simulink model "Simulation_NoVI"  (R2022b)
settings: Solver=VariableStepAuto  StartTime=0.0  StopTime=25  RelTol=1e-3
values from neighbouring files (symbols this model uses):
  A = [0 1 1 1 ; 1 0 1 1 ; 1 1 0 1 ; 1 1 1 0]    [Primary_test1.m]    (also in init.mat = [0 1 1 1 1 0 1 1 1 1 0 1 ... (16 elements, 4x4)])
  C_f = 0.000112315*9    (= 0.001010835)    [Main.m]    (also in PSO_2paras.m = swarm(i,2); PSO_filter_2paras.m = swarm(i,2)/10000; Primary_test1.m; Script_18June.m = 0.0112315)
  f_c = 50e3    (= 50000)    [Main.m]    (also in Primary_test1.m; Script_18June.m; Script_23June.m; Script_5thJune.m)
  k = -0.5    [Main.m]    (also in Primary_test1.m; Savedata.m = 0.2909; Script_18June.m = 0.5; Script_23June.m)
  K_h11 = 0    [Main.m]    (also in PSO_HC.m = swarm(i,4); Primary_test1.m; Script_18June.m; Script_23June.m)
  K_h13 = 0    [Main.m]    (also in Primary_test1.m; Script_18June.m; Script_23June.m; Script_5thJune.m)
  K_h5 = 0    [Main.m]    (also in PSO_HC.m = swarm(i,1); Primary_test1.m = 1; Script_18June.m; Script_23June.m)
  K_h7 = 0    [Main.m]    (also in PSO_HC.m = swarm(i,2); Primary_test1.m; Script_18June.m; Script_23June.m)
  K_h9 = 0    [Main.m]    (also in PSO_HC.m = swarm(i,3); Script_18June.m; Script_23June.m; Script_5thJune.m)
  ki_pr = 160    [Main.m]    (also in PSO.m = swarm(i,2); Primary_test1.m; Savedata.m = 422.4716; Script_18June.m = 150)
  kL = 1e-7    (= 1e-07)    [Main.m]    (also in Primary_test1.m; Script_18June.m; Script_23June.m; Script_5thJune.m)
  Kp_pr = 1.7    [Main.m]    (also in PSO.m = swarm(i,1); Primary_test1.m; Savedata.m = 0.9028; Script_18June.m = 1)
  L_f = 0.000659829*1.4    (= 0.0009237606)    [Main.m]    (also in PSO_2paras.m = swarm(i,1); PSO_filter_2paras.m = swarm(i,1); Primary_test1.m; Script_18June.m = 0.000295603392)
  L_in1 = 0.35e-3    (= 0.00035)    [Main.m]    (also in Primary_test1.m; Script_18June.m; Script_23June.m; Script_5thJune.m)
  L_in2 = 0.35e-3    (= 0.00035)    [Main.m]    (also in Primary_test1.m; Script_18June.m; Script_23June.m; Script_5thJune.m)
  L_in3 = 0.35e-3    (= 0.00035)    [Main.m]    (also in Primary_test1.m; Script_18June.m; Script_23June.m; Script_5thJune.m)
  L_in4 = 0.35e-3    (= 0.00035)    [Main.m]    (also in Primary_test1.m; Script_18June.m; Script_23June.m; Script_5thJune.m)
  lambda1 = 5.5*[1 1 0.8 0.8]'    [Primary_test1.m]    (also in init.mat = [5.5 5.5 4.4 4.4])
  lambda2 = 30.5*[0.8e-2 0.8e-2 0.5e-2 0.5e-2]'    [Primary_test1.m]    (also in init.mat = [0.244 0.244 0.1525 0.1525])
  lambda3 = 62.5*[1.5e-3 1.5e-3 1e-3 1.1e-3]'    [Primary_test1.m]    (also in init.mat = [0.09375 0.09375 0.0625 0.06875])
  LD_ref1 = 100e-6    (= 0.0001)    [Main.m]    (also in Primary_test1.m; Script_18June.m = 5e-05; Script_23June.m = 1e-05; Script_5thJune.m = 1e-05)
  lo_co = 0.1    [Main.m]    (also in Primary_test1.m; Script_18June.m; Script_23June.m; Script_5thJune.m)
  load_off = 10    [Main.m]    (also in Primary_test1.m = 2; Script_18June.m = 28; Script_23June.m = 28; Script_5thJune.m)
  load_on = 0.21    [Main.m]    (also in Primary_test1.m = 1; Script_18June.m; Script_23June.m; Script_5thJune.m)
  m_p1 = 9.4e-5/droopDivide    (= 9.4e-06)    [Main.m]    (also in Primary_test1.m; Script_18June.m = 9.4e-05; Script_23June.m = 9.4e-05; Script_5thJune.m = 5e-05)
  m_p2 = 9.4e-5/droopDivide    (= 9.4e-06)    [Main.m]    (also in Primary_test1.m; Script_18June.m = 9.4e-05; Script_23June.m = 9.4e-05; Script_5thJune.m = 5e-05)
  m_p3 = 11.4e-5/droopDivide    (= 1.14e-05)    [Main.m]    (also in Primary_test1.m; Script_18June.m = 0.000114; Script_23June.m = 0.000114; Script_5thJune.m = 6.42857142857e-05)
  m_p4 = 11.4e-5/droopDivide    (= 1.14e-05)    [Main.m]    (also in Primary_test1.m; Script_18June.m = 0.000114; Script_23June.m = 0.000114; Script_5thJune.m = 6.42857142857e-05)
  N = 2    [Primary_test1.m]    (also in init.mat)
  n_q1 = 1.3e-3/droopDivide2    (= 6.5e-05)    [Main.m]    (also in Primary_test1.m; Script_18June.m; Script_23June.m; Script_5thJune.m = 0.2)
  n_q2 = 1.3e-3/droopDivide2    (= 6.5e-05)    [Main.m]    (also in Primary_test1.m; Script_18June.m; Script_23June.m; Script_5thJune.m = 0.2)
  n_q3 = 1.5e-3/droopDivide2    (= 7.5e-05)    [Main.m]    (also in Primary_test1.m; Script_18June.m; Script_23June.m; Script_5thJune.m = 0.257142857143)
  n_q4 = 1.5e-3/droopDivide2    (= 7.5e-05)    [Main.m]    (also in Primary_test1.m; Script_18June.m; Script_23June.m; Script_5thJune.m = 0.257142857143)
  Pmax = [45e3 45e3 37e3 37e3]'    [Primary_test1.m]    (also in init.mat = [45000 45000 37000 37000])
  PMW = V_nom/0.55    [Main.m]    (also in Primary_test1.m; Script_18June.m = V_nom/0.4; Script_23June.m; Script_5thJune.m = 220*sqrt(2))
  R_f = 0.35    [Main.m]    (also in PSO_filter_2paras.m = 10*L_f; Primary_test1.m; Savedata.m = 0.249593207053; Script_18June.m = 0.1)
  R_in1 = 0.03    [Main.m]    (also in Primary_test1.m; Script_18June.m; Script_23June.m; Script_5thJune.m)
  R_in2 = 0.03    [Main.m]    (also in Primary_test1.m; Script_18June.m; Script_23June.m; Script_5thJune.m)
  R_in3 = 0.03    [Main.m]    (also in Primary_test1.m; Script_18June.m; Script_23June.m; Script_5thJune.m)
  R_in4 = 0.03    [Main.m]    (also in Primary_test1.m; Script_18June.m; Script_23June.m; Script_5thJune.m)
  time_thresh = 0.2    [Main.m]    (also in Primary_test1.m; Script_18June.m; Script_23June.m; Script_5thJune.m)
  Ts = 10e-6    (= 1e-05)    [Main.m]    (also in Primary_test1.m; Script_18June.m; Script_23June.m; Script_5thJune.m)
  Tsamp = 0.1    [Primary_test1.m]    (also in init.mat)
  V_nom = 220*sqrt(2)    [Main.m]    (also in Primary_test1.m; Script_18June.m; Script_23June.m; Script_5thJune.m)
  Vdc = 600    [Main.m]    (also in Primary_test1.m; Script_18June.m; Script_23June.m; Script_5thJune.m)
  w_c_high = 2*pi*50    (= 314.159265359)    [Main.m]    (also in Primary_test1.m; Script_18June.m = 307.876080052; Script_23June.m; Script_5thJune.m = 307.876080052)
  w_nom = 2*pi*f    (= 314.159265359)    [Main.m]    (also in Primary_test1.m; Script_18June.m; Script_23June.m; Script_5thJune.m)
  wc_hc = 1    [Main.m]    (also in Primary_test1.m; Script_18June.m = 0.3; Script_23June.m; Script_5thJune.m = 0.3)
  wc_pr = 3    [Main.m]    (also in PSO.m = swarm(i,3); Primary_test1.m; Savedata.m = 1.36672; Script_18June.m = 1.5)
undefined symbols (not defined in the file or in its folder): DiscIntNeverNeededParam, i
libraries: eeGeneralControl x16, spsThreePhaseSeriesRLCBranchLib x15, spsThreePhaseVIMeasurementLib x12, spsabctoAlphaBetaZeroLib x12, spsabctodq0Lib x12, slpidlib x8, spsThreePhaseSeriesRLCLoadLib x6, spsThreePhaseBreakerLib x6, spsDCVoltageSourceLib x4, spsAlphaBetaZerotoabcLib x4, spsSeriesRLCBranchLib x4, spsTriangleGeneratorLib x4
(part 3 of 5)

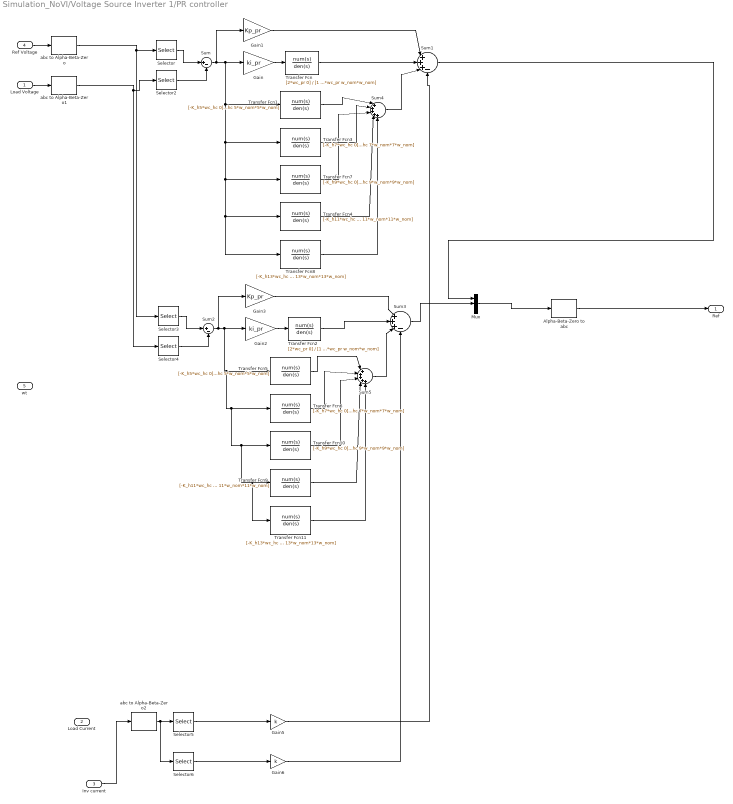
== system Simulation_NoVI/Voltage Source Inverter 1/PR controller ==
  Load Voltage : Inport
  Load Current : Inport  Port=2
  Inv current : Inport  Port=3
  Ref Voltage : Inport  Port=4
  wt : Inport  Port=5
  Alpha-Beta-Zero to abc : spsAlphaBetaZerotoabcLib/Alpha-Beta-Zero to abc
      settings: LibrarySourceBlock=|
      | sps_lib/Control/Alpha-Beta-Zero
      | to abc
  Gain : Gain  Gain=ki_pr
  Gain1 : Gain  Gain=Kp_pr
  Gain2 : Gain  Gain=ki_pr
  Gain3 : Gain  Gain=Kp_pr
  Gain5 : Gain  Gain=k
  Gain6 : Gain  Gain=k
  Mux : Mux  Inputs=3
  Selector : Selector  InputPortWidth=3  IndexOptions=Index vector (dialog)  Indices=[1]  OutputSizes=1
  Selector2 : Selector  InputPortWidth=3  IndexOptions=Index vector (dialog)  Indices=[1]  OutputSizes=1
  Selector3 : Selector  InputPortWidth=3  IndexOptions=Index vector (dialog)  Indices=[2]  OutputSizes=1
  Selector4 : Selector  InputPortWidth=3  IndexOptions=Index vector (dialog)  Indices=[2]  OutputSizes=1
  Selector5 : Selector  InputPortWidth=3  IndexOptions=Index vector (dialog)  Indices=[1]  OutputSizes=1
  Selector6 : Selector  InputPortWidth=3  IndexOptions=Index vector (dialog)  Indices=[2]  OutputSizes=1
  Sum : Sum  Inputs=|+-
  Sum1 : Sum  Inputs=|+++-
  Sum2 : Sum  Inputs=|+-
  Sum3 : Sum  Inputs=|+++-
  Sum4 : Sum  Inputs=|+++++
  Sum5 : Sum  Inputs=|+++++
  Transfer Fcn : TransferFcn  Numerator=[2*wc_pr 0]  Denominator=[1 2*wc_pr*wc_pr w_nom*w_nom]
  Transfer Fcn1 : TransferFcn  Numerator=[-K_h5*wc_hc 0]  Denominator=[1 2*wc_hc 5*w_nom*5*w_nom]
  Transfer Fcn10 : TransferFcn  Numerator=[-K_h9*wc_hc 0]  Denominator=[1 2*wc_hc 9*w_nom*9*w_nom]
  Transfer Fcn11 : TransferFcn  Numerator=[-K_h13*wc_hc 0]  Denominator=[1 2*wc_hc 13*w_nom*13*w_nom]
  Transfer Fcn2 : TransferFcn  Numerator=[2*wc_pr 0]  Denominator=[1 2*wc_pr*wc_pr w_nom*w_nom]
  Transfer Fcn3 : TransferFcn  Numerator=[-K_h7*wc_hc 0]  Denominator=[1 2*wc_hc 7*w_nom*7*w_nom]
  Transfer Fcn4 : TransferFcn  Numerator=[-K_h11*wc_hc 0]  Denominator=[1 2*wc_hc 11*w_nom*11*w_nom]
  Transfer Fcn5 : TransferFcn  Numerator=[-K_h5*wc_hc 0]  Denominator=[1 2*wc_hc 5*w_nom*5*w_nom]
  Transfer Fcn6 : TransferFcn  Numerator=[-K_h7*wc_hc 0]  Denominator=[1 2*wc_hc 7*w_nom*7*w_nom]
  Transfer Fcn7 : TransferFcn  Numerator=[-K_h9*wc_hc 0]  Denominator=[1 2*wc_hc 9*w_nom*9*w_nom]
  Transfer Fcn8 : TransferFcn  Numerator=[-K_h13*wc_hc 0]  Denominator=[1 2*wc_hc 13*w_nom*13*w_nom]
  Transfer Fcn9 : TransferFcn  Numerator=[-K_h11*wc_hc 0]  Denominator=[1 2*wc_hc 11*w_nom*11*w_nom]
  abc to Alpha-Beta-Zero : spsabctoAlphaBetaZeroLib/abc to Alpha-Beta-Zero
  abc to Alpha-Beta-Zero1 : spsabctoAlphaBetaZeroLib/abc to Alpha-Beta-Zero
  abc to Alpha-Beta-Zero2 : spsabctoAlphaBetaZeroLib/abc to Alpha-Beta-Zero
  Ref : Outport
  wires:
  Ref Voltage/1 -> abc to Alpha-Beta-Zero/1
  Selector/1 -> Sum/1
  Selector2/1 -> Sum/2
  Sum/1 -> Gain1/1, Transfer Fcn8/1, Transfer Fcn4/1, Transfer Fcn7/1, Transfer Fcn3/1, Transfer Fcn1/1, Gain/1
  Gain/1 -> Transfer Fcn/1
  Gain1/1 -> Sum1/1
  Transfer Fcn/1 -> Sum1/2
  Sum2/1 -> Gain3/1, Transfer Fcn11/1, Transfer Fcn9/1, Transfer Fcn10/1, Transfer Fcn6/1, Transfer Fcn5/1, Gain2/1
  Selector3/1 -> Sum2/1
  Gain2/1 -> Transfer Fcn2/1
  Transfer Fcn2/1 -> Sum3/2
  Gain3/1 -> Sum3/1
  abc to Alpha-Beta-Zero2/1 -> Selector6/1, Selector5/1
  Sum1/1 -> Mux/1
  Sum3/1 -> Mux/2
  Mux/1 -> Alpha-Beta-Zero to abc/1
  Inv current/1 -> abc to Alpha-Beta-Zero2/1
  Sum4/1 -> Sum1/3
  Transfer Fcn1/1 -> Sum4/1
  Transfer Fcn3/1 -> Sum4/2
  Transfer Fcn6/1 -> Sum5/2
  Selector4/1 -> Sum2/2
  Sum5/1 -> Sum3/3
  Transfer Fcn7/1 -> Sum4/3
  Transfer Fcn4/1 -> Sum4/4
  Transfer Fcn8/1 -> Sum4/5
  Transfer Fcn10/1 -> Sum5/3
  Transfer Fcn9/1 -> Sum5/4
  Transfer Fcn11/1 -> Sum5/5
  Selector6/1 -> Gain6/1
  Selector5/1 -> Gain5/1
  Transfer Fcn5/1 -> Sum5/1
  Gain5/1 -> Sum1/4
  Gain6/1 -> Sum3/4
  Load Voltage/1 -> abc to Alpha-Beta-Zero1/1
  abc to Alpha-Beta-Zero/1 -> Selector3/1, Selector/1
  abc to Alpha-Beta-Zero1/1 -> Selector4/1, Selector2/1
  Alpha-Beta-Zero to abc/1 -> Ref/1

== system Simulation_NoVI/Voltage Source Inverter 1/dq converter ==
  Vodq : Inport
  Iodq : Inport  Port=2
  Ildq : Inport  Port=3
  wt : Inport  Port=4
  Scope : Scope
  Scope1 : Scope
  Subsystem : Subsystem
  Subsystem1 : Subsystem
  Subsystem2 : Subsystem
  Vod : Outport
  Voq : Outport  Port=2
  Iod : Outport  Port=3
  Ioq : Outport  Port=4
  Ild : Outport  Port=5
  Ilq : Outport  Port=6
  wires:
  Subsystem/1(Out1) -> Scope/1, Vod/1  "Vod"
  Subsystem1/1(Out1) -> Iod/1  "Iod"
  Subsystem/2(Out2) -> Voq/1  "Voq"
  wt/1 -> Subsystem2/2(wt), Subsystem1/2(wt), Subsystem/2(wt)
  Subsystem1/2(Out2) -> Ioq/1  "Ioq"
  Iodq/1 -> Subsystem1/1(abc)
  Subsystem2/2(Out2) -> Ilq/1  "Ilq"
  Ildq/1 -> Subsystem2/1(abc)
  Vodq/1 -> Subsystem/1(abc)
  Subsystem2/1(Out1) -> Scope1/1, Ild/1  "Vod"

== system Simulation_NoVI/Voltage Source Inverter 2/3to2 3 ==
  "single " : Inport
  "wt " : Inport  Port=2
  Add1 : Sum  Inputs=+++
  Constant2 : Constant  Value=2*pi/3
  Constant3 : Constant  Value=4*pi/3
  Constant4 : Constant  Value=exp(i*2*pi/3)
  Constant5 : Constant  Value=2/3
  Cos : Trigonometry  Operator=cos
  Cos1 : Trigonometry  Operator=cos
  Cos2 : Trigonometry  Operator=cos
  Math Function1 : Math  Operator=square  SignedPower=on
  Mux : Mux  Inputs=3
  Product{3..8} (6 alike) : Product  RndMeth=Zero
  Scope : Scope  NumInputPorts=3
  Sum : Sum  Inputs=|++
  Sum1 : Sum  Inputs=|++
  threePhase : Outport  VectorParamsAs1DForOutWhenUnconnected=off
  wires:
  "single "/1 -> Product5/1, Product4/1, Product3/1
  Cos/1 -> Product3/2
  Constant2/1 -> Sum/2
  Sum/1 -> Cos1/1
  Cos1/1 -> Product4/2
  "wt "/1 -> Sum1/1, Sum/1, Cos/1
  Constant3/1 -> Sum1/2
  Sum1/1 -> Cos2/1
  Cos2/1 -> Product5/2
  Constant4/1 -> Product7/1, Math Function1/1
  Product7/1 -> Add1/2
  Add1/1 -> Product6/1
  Product8/1 -> Add1/3
  Product5/1 -> Scope/3, Mux/3, Product8/2
  Product3/1 -> Scope/1, Mux/1, Add1/1
  Constant5/1 -> Product6/2
  Product4/1 -> Scope/2, Mux/2, Product7/2
  Math Function1/1 -> Product8/1
  Mux/1 -> threePhase/1

== system Simulation_NoVI/Voltage Source Inverter 2/Droop for secondary control2 ==
  P : Inport
  w_nom : Inport  Port=2
  V_nom : Inport  Port=3
  Q : Inport  Port=4
  Gain4 : Gain  Gain=n_q
  Gain5 : Gain  Gain=m_p
  Integrator : Integrator  WrapState=on  WrappedStateUpperValue=2*pi  WrappedStateLowerValue=0
  Sum1 : Sum  Inputs=|+-
  Sum2 : Sum  Inputs=|+-
  Vref : Outport
  wt : Outport  Port=2
  wo : Outport  Port=3
  wires:
  P/1 -> Gain5/1
  w_nom/1 -> Sum2/1
  Gain5/1 -> Sum2/2
  Sum2/1 -> wo/1, Integrator/1  "w"
  Integrator/1 -> wt/1
  V_nom/1 -> Sum1/1  "Vod_s"
  Gain4/1 -> Sum1/2
  Q/1 -> Gain4/1
  Sum1/1 -> Vref/1  "Vod_s"

== system Simulation_NoVI/Voltage Source Inverter 2/Low-pass filter ==
  p_hat : Inport
  q_hat : Inport  Port=2
  Low-Pass Filter (Discrete or Continuous) : eeGeneralControl/Low-Pass Filter (Discrete or Continuous)  K=1  T=lo_co  B=inf  A=-inf  init_option=Inherited from block input  x0=0  Ts=-1
  Low-Pass Filter (Discrete or Continuous)1 : eeGeneralControl/Low-Pass Filter (Discrete or Continuous)  K=1  T=lo_co  B=inf  A=-inf  init_option=Inherited from block input  x0=0  Ts=-1
  P : Outport
  Q : Outport  Port=2
  wires:
  q_hat/1 -> Low-Pass Filter (Discrete or Continuous)1/1
  Low-Pass Filter (Discrete or Continuous)1/1 -> Q/1  "Q"
  Low-Pass Filter (Discrete or Continuous)/1 -> P/1  "P"
  p_hat/1 -> Low-Pass Filter (Discrete or Continuous)/1

== system Simulation_NoVI/Voltage Source Inverter 2/PLL_1p1 ==
  v : Inport
  2pi : Constant  Value=2*pi
  Low-Pass Filter (Discrete or Continuous) : eeGeneralControl/Low-Pass Filter (Discrete or Continuous)  K=1  T=lo_co  B=inf  A=-inf  init_option=Inherited from block input  x0=0  Ts=-1
  PID Controller : slpidlib/PID Controller  Controller=PI  Form=Parallel  TimeDomain=Continuous-time  UseExternalTs=off  SampleTime=-1  IntegratorMethod=Forward Euler  FilterMethod=Forward Euler  ControllerParametersSource=internal  P=100.15925  I=9869  UseKiTs=off  D=0  N=100  UseFilter=on  TunerSelectOption=Transfer Function Based (PID Tuner App)  InitialConditionSource=internal  InitialConditionForIntegrator=0  InitialConditionForFilter=0  DifferentiatorICPrevScaledInput=0  ExternalReset=none  TrackingMode=off  Kt=1  LimitOutput=off  SatLimitsSource=internal  UpperSaturationLimit=inf  LowerSaturationLimit=-inf  LinearizeAsGain=off  AntiWindupMode=none  Kb=1  LimitIntegrator=off  UpperIntegratorSaturationLimit=inf  LowerIntegratorSaturationLimit=-inf  POutMin=[]  POutMax=[]  IOutMin=[]  IOutMax=[]  DOutMin=[]  DOutMax=[]  NOutMin=[]  NOutMax=[]  SumOutMin=[]  SumOutMax=[]  SaturationOutMin=[]  SaturationOutMax=[]  PParamMin=[]  PParamMax=[]  IParamMin=[]  IParamMax=[]  DParamMin=[]  DParamMax=[]  NParamMin=[]  NParamMax=[]  KbParamMin=[]  KbParamMax=[]  KtParamMin=[]  KtParamMax=[]  KbOutMin=[]  KbOutMax=[]  KtOutMin=[]  KtOutMax=[]  IntegratorOutMin=[]  IntegratorOutMax=[]  FilterOutMin=[]  FilterOutMax=[]  SumI1OutMin=[]  SumI1OutMax=[]  SumI2OutMin=[]  SumI2OutMax=[]  SumI3OutMin=[]  SumI3OutMax=[]  SumI4OutMin=[]  SumI4OutMax=[]  SumDOutMin=[]  SumDOutMax=[]  DifferentiatorOutMin=[]  DifferentiatorOutMax=[]  FilterDiffOutCoefMin=[]  FilterDiffOutCoefMax=[]  ReciprocalOutMin=[]  ReciprocalOutMax=[]  SumDenOutMin=[]  SumDenOutMax=[]  SumNumOutMin=[]  SumNumOutMax=[]  DivideOutMin=[]  DivideOutMax=[]  UdiffTsProdOutMin=[]  UdiffTsProdOutMax=[]  NTsProdOutMin=[]  NTsProdOutMax=[]  UintegralTsProdOutMin=[]  UintegralTsProdOutMax=[]  UngainTsProdOutMin=[]  UngainTsProdOutMax=[]  ClampingZeroOutDataTypeStr=Inherit: Inherit via back propagation  ClampingZeroOutMin=[]  ClampingZeroOutMax=[]  FilterDenConstantOutDataTypeStr=Inherit: Inherit via back propagation  FilterDenConstantOutMin=[]  FilterDenConstantOutMax=[]  PCopyOutDataTypeStr=Inherit: Inherit via back propagation  PCopyOutMin=[]  PCopyOutMax=[]  NCopyOutDataTypeStr=Inherit: Inherit via back propagation  NCopyOutMin=[]  NCopyOutMax=[]  IntegratorContinuousStateAttributes=''  IntegratorStateMustResolveToSignalObject=off  IntegratorRTWStateStorageClass=Auto  FilterContinuousStateAttributes=''  FilterStateMustResolveToSignalObject=off  FilterRTWStateStorageClass=Auto  ParallelPVariant=InternalParameters  IdealPVariant=Disabled  IVariant=InternalParameters  DVariant=Disabled  IntegratorVariant=Continuous  SatVariant=Disabled  AWVariant=Passthrough  PCopyVariant=Disabled  TRVariant=Disabled  FdbkBlocksVariant=Forward  IdealPFdbkVariant=Disabled  SatFdbkVariant=Disabled  DerivativeFilterVariant=Disabled  NVariant=Disabled  NCopyVariant=Disabled_SignalSpec  FilterICVariant=Disabled  IntegratorICVariant=InternalICs  ExternalResetVariant=Disabled  TRSumVariant=Passthrough  SumFdbkVariant=Disabled  SumVariant=Sum_PI  TsampFilterVariant=InternalTs  TsampNgainVariant=Passthrough  TsampIntegralVariant=Passthrough  ExternalSaturationOutDataTypeStr=Inherit: Same as second input
  Reset1 : RelationalOperator  OutDataTypeStr=boolean  InputSameDT=off
  Scope : Scope
  Sqrt : Sqrt
  Square : Math  Operator=square
  Square1 : Math  Operator=square
  Sum : Sum  Inputs=|++
  Sum1 : Sum  Inputs=|++
  TienXuly : Subsystem  mask{k=0.5, fc1=50, fc2=10}
      mask prompts: k "he so k"; fc1 "Tan so cat cua bo loc bac 2"; fc2 "Tan so cat cua bo loc thong thap"
  Tinhtheta : Integrator  ExternalReset=rising  UpperSaturationLimit=2*pi
  apha-beta=>dq : Subsystem
  wff : Constant  Value=50*2*pi
  v_dq : Outport
  omega : Outport  Port=2
  wires:
  PID Controller/1 -> Sum1/1
  v/1 -> TienXuly/1(v)
  Tinhtheta/1 -> apha-beta=>dq/1(Theta), Reset1/1
  TienXuly/2(v'q) -> apha-beta=>dq/3(Ubeta)
  apha-beta=>dq/1(vq) -> Square1/1, PID Controller/1
  TienXuly/1(v') -> apha-beta=>dq/2(Uapha)
  2pi/1 -> Reset1/2
  wff/1 -> Sum1/2
  Reset1/1 -> Tinhtheta/2
  apha-beta=>dq/2(vd) -> Square/1
  Square/1 -> Sum/1
  Square1/1 -> Sum/2
  Sum/1 -> Sqrt/1
  Sqrt/1 -> v_dq/1
  Sum1/1 -> Low-Pass Filter (Discrete or Continuous)/1, Tinhtheta/1  "P"
  Low-Pass Filter (Discrete or Continuous)/1 -> Scope/1, omega/1  "P"

== system Simulation_NoVI/Voltage Source Inverter 2/PLL_1p2 ==
  v : Inport
  2pi : Constant  Value=2*pi
  Low-Pass Filter (Discrete or Continuous) : eeGeneralControl/Low-Pass Filter (Discrete or Continuous)  K=1  T=lo_co  B=inf  A=-inf  init_option=Inherited from block input  x0=0  Ts=-1
  PID Controller : slpidlib/PID Controller  Controller=PI  Form=Parallel  TimeDomain=Continuous-time  UseExternalTs=off  SampleTime=-1  IntegratorMethod=Forward Euler  FilterMethod=Forward Euler  ControllerParametersSource=internal  P=100.15925  I=9869  UseKiTs=off  D=0  N=100  UseFilter=on  TunerSelectOption=Transfer Function Based (PID Tuner App)  InitialConditionSource=internal  InitialConditionForIntegrator=0  InitialConditionForFilter=0  DifferentiatorICPrevScaledInput=0  ExternalReset=none  TrackingMode=off  Kt=1  LimitOutput=off  SatLimitsSource=internal  UpperSaturationLimit=inf  LowerSaturationLimit=-inf  LinearizeAsGain=off  AntiWindupMode=none  Kb=1  LimitIntegrator=off  UpperIntegratorSaturationLimit=inf  LowerIntegratorSaturationLimit=-inf  POutMin=[]  POutMax=[]  IOutMin=[]  IOutMax=[]  DOutMin=[]  DOutMax=[]  NOutMin=[]  NOutMax=[]  SumOutMin=[]  SumOutMax=[]  SaturationOutMin=[]  SaturationOutMax=[]  PParamMin=[]  PParamMax=[]  IParamMin=[]  IParamMax=[]  DParamMin=[]  DParamMax=[]  NParamMin=[]  NParamMax=[]  KbParamMin=[]  KbParamMax=[]  KtParamMin=[]  KtParamMax=[]  KbOutMin=[]  KbOutMax=[]  KtOutMin=[]  KtOutMax=[]  IntegratorOutMin=[]  IntegratorOutMax=[]  FilterOutMin=[]  FilterOutMax=[]  SumI1OutMin=[]  SumI1OutMax=[]  SumI2OutMin=[]  SumI2OutMax=[]  SumI3OutMin=[]  SumI3OutMax=[]  SumI4OutMin=[]  SumI4OutMax=[]  SumDOutMin=[]  SumDOutMax=[]  DifferentiatorOutMin=[]  DifferentiatorOutMax=[]  FilterDiffOutCoefMin=[]  FilterDiffOutCoefMax=[]  ReciprocalOutMin=[]  ReciprocalOutMax=[]  SumDenOutMin=[]  SumDenOutMax=[]  SumNumOutMin=[]  SumNumOutMax=[]  DivideOutMin=[]  DivideOutMax=[]  UdiffTsProdOutMin=[]  UdiffTsProdOutMax=[]  NTsProdOutMin=[]  NTsProdOutMax=[]  UintegralTsProdOutMin=[]  UintegralTsProdOutMax=[]  UngainTsProdOutMin=[]  UngainTsProdOutMax=[]  ClampingZeroOutDataTypeStr=Inherit: Inherit via back propagation  ClampingZeroOutMin=[]  ClampingZeroOutMax=[]  FilterDenConstantOutDataTypeStr=Inherit: Inherit via back propagation  FilterDenConstantOutMin=[]  FilterDenConstantOutMax=[]  PCopyOutDataTypeStr=Inherit: Inherit via back propagation  PCopyOutMin=[]  PCopyOutMax=[]  NCopyOutDataTypeStr=Inherit: Inherit via back propagation  NCopyOutMin=[]  NCopyOutMax=[]  IntegratorContinuousStateAttributes=''  IntegratorStateMustResolveToSignalObject=off  IntegratorRTWStateStorageClass=Auto  FilterContinuousStateAttributes=''  FilterStateMustResolveToSignalObject=off  FilterRTWStateStorageClass=Auto  ParallelPVariant=InternalParameters  IdealPVariant=Disabled  IVariant=InternalParameters  DVariant=Disabled  IntegratorVariant=Continuous  SatVariant=Disabled  AWVariant=Passthrough  PCopyVariant=Disabled  TRVariant=Disabled  FdbkBlocksVariant=Forward  IdealPFdbkVariant=Disabled  SatFdbkVariant=Disabled  DerivativeFilterVariant=Disabled  NVariant=Disabled  NCopyVariant=Disabled_SignalSpec  FilterICVariant=Disabled  IntegratorICVariant=InternalICs  ExternalResetVariant=Disabled  TRSumVariant=Passthrough  SumFdbkVariant=Disabled  SumVariant=Sum_PI  TsampFilterVariant=InternalTs  TsampNgainVariant=Passthrough  TsampIntegralVariant=Passthrough  ExternalSaturationOutDataTypeStr=Inherit: Same as second input
  Reset1 : RelationalOperator  OutDataTypeStr=boolean  InputSameDT=off
  Scope : Scope
  Sqrt : Sqrt
  Square : Math  Operator=square
  Square1 : Math  Operator=square
  Sum : Sum  Inputs=|++
  Sum1 : Sum  Inputs=|++
  TienXuly : Subsystem  mask{k=0.5, fc1=50, fc2=10}
      mask prompts: k "he so k"; fc1 "Tan so cat cua bo loc bac 2"; fc2 "Tan so cat cua bo loc thong thap"
  Tinhtheta : Integrator  ExternalReset=rising  UpperSaturationLimit=2*pi
  apha-beta=>dq : Subsystem
  wff : Constant  Value=50*2*pi
  v_dq : Outport
  omega : Outport  Port=2
  wires:
  PID Controller/1 -> Sum1/1
  v/1 -> TienXuly/1(v)
  Tinhtheta/1 -> apha-beta=>dq/1(Theta), Reset1/1
  TienXuly/2(v'q) -> apha-beta=>dq/3(Ubeta)
  apha-beta=>dq/1(vq) -> Square1/1, PID Controller/1
  TienXuly/1(v') -> apha-beta=>dq/2(Uapha)
  2pi/1 -> Reset1/2
  wff/1 -> Sum1/2
  Reset1/1 -> Tinhtheta/2
  apha-beta=>dq/2(vd) -> Square/1
  Square/1 -> Sum/1
  Square1/1 -> Sum/2
  Sum/1 -> Sqrt/1
  Sqrt/1 -> v_dq/1
  Sum1/1 -> Low-Pass Filter (Discrete or Continuous)/1, Tinhtheta/1  "P"
  Low-Pass Filter (Discrete or Continuous)/1 -> Scope/1, omega/1  "P"

== system Simulation_NoVI/Voltage Source Inverter 2/PMW ==
  REF : Inport
  Tri_signal : Inport  Port=2
  Demux : Demux  Outputs=3
  Mux : Mux  Inputs=6
  NOT : Logic  Operator=NOT  AllPortsSameDT=off  OutDataTypeStr=boolean
  NOT1 : Logic  Operator=NOT  AllPortsSameDT=off  OutDataTypeStr=boolean
  NOT2 : Logic  Operator=NOT  AllPortsSameDT=off  OutDataTypeStr=boolean
  Relational Operator : RelationalOperator  OutDataTypeStr=boolean  RndMeth=Simplest  InputSameDT=off
  Relational Operator1 : RelationalOperator  OutDataTypeStr=boolean  RndMeth=Simplest  InputSameDT=off
  Relational Operator2 : RelationalOperator  OutDataTypeStr=boolean  RndMeth=Simplest  InputSameDT=off
  Scope : Scope
  Scope1 : Scope
  Scope2 : Scope  NumInputPorts=2
  Out1 : Outport
  wires:
  Demux/1 -> Relational Operator/1
  Tri_signal/1 -> Relational Operator1/2, Relational Operator/2, Relational Operator2/2
  Demux/2 -> Relational Operator1/1
  Demux/3 -> Relational Operator2/1
  REF/1 -> Scope1/1, Demux/1
  Relational Operator/1 -> Scope2/1, Mux/1, NOT/1
  NOT/1 -> Scope2/2, Mux/2
  Relational Operator1/1 -> NOT1/1, Mux/3
  NOT1/1 -> Mux/4
  Relational Operator2/1 -> Mux/5, NOT2/1
  NOT2/1 -> Mux/6
  Mux/1 -> Scope/1, Out1/1

== system Simulation_NoVI/Voltage Source Inverter 2/PQ calculator ==
  Vod : Inport
  Voq : Inport  Port=2
  Iod : Inport  Port=3
  Ioq : Inport  Port=4
  Product{,1..3} (4 alike) : Product
  Scope : Scope
  Sum10 : Sum  Inputs=|++
  Sum11 : Sum  Inputs=|+-
  p_hat : Outport
  q_hat : Outport  Port=2
  wires:
  Product3/1 -> Sum11/2
  Product1/1 -> Sum10/2
  Voq/1 -> Product3/1, Product1/1
  Iod/1 -> Product/2, Product3/2
  Product2/1 -> Sum11/1
  Ioq/1 -> Product1/2, Product2/2
  Product/1 -> Sum10/1
  Vod/1 -> Scope/1, Product/1, Product2/1
  Sum11/1 -> q_hat/1  "q_hat"
  Sum10/1 -> p_hat/1  "p_hat"

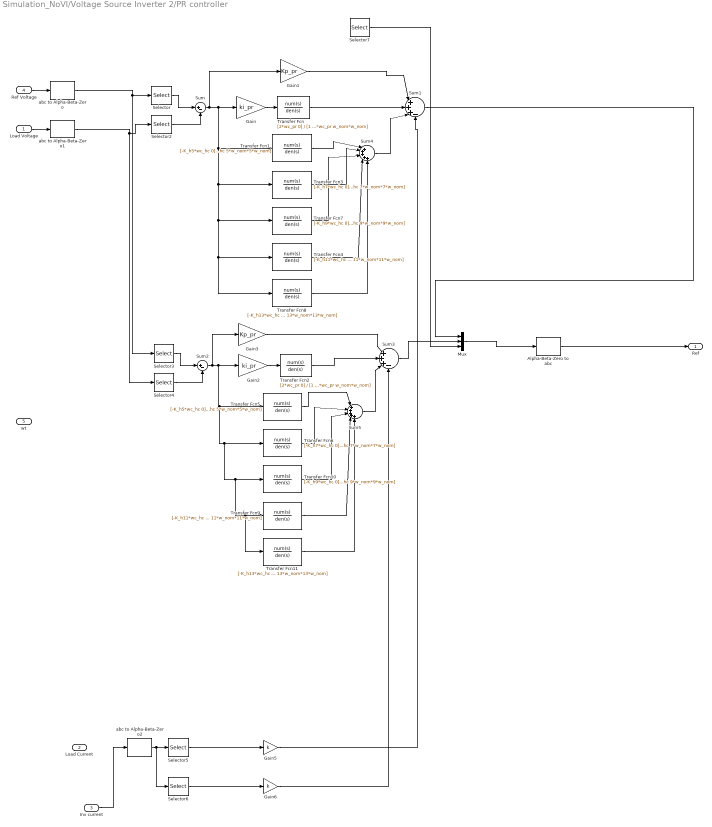
== system Simulation_NoVI/Voltage Source Inverter 2/PR controller ==
  Load Voltage : Inport
  Load Current : Inport  Port=2
  Inv current : Inport  Port=3
  Ref Voltage : Inport  Port=4
  wt : Inport  Port=5
  Alpha-Beta-Zero to abc : spsAlphaBetaZerotoabcLib/Alpha-Beta-Zero to abc
      settings: LibrarySourceBlock=|
      | sps_lib/Control/Alpha-Beta-Zero
      | to abc
  Gain : Gain  Gain=ki_pr
  Gain1 : Gain  Gain=Kp_pr
  Gain2 : Gain  Gain=ki_pr
  Gain3 : Gain  Gain=Kp_pr
  Gain5 : Gain  Gain=k
  Gain6 : Gain  Gain=k
  Mux : Mux  Inputs=3
  Selector : Selector  InputPortWidth=3  IndexOptions=Index vector (dialog)  Indices=[1]  OutputSizes=1
  Selector2 : Selector  InputPortWidth=3  IndexOptions=Index vector (dialog)  Indices=[1]  OutputSizes=1
  Selector3 : Selector  InputPortWidth=3  IndexOptions=Index vector (dialog)  Indices=[2]  OutputSizes=1
  Selector4 : Selector  InputPortWidth=3  IndexOptions=Index vector (dialog)  Indices=[2]  OutputSizes=1
  Selector5 : Selector  InputPortWidth=3  IndexOptions=Index vector (dialog)  Indices=[1]  OutputSizes=1
  Selector6 : Selector  InputPortWidth=3  IndexOptions=Index vector (dialog)  Indices=[2]  OutputSizes=1
  Selector7 : Selector  InputPortWidth=3  IndexOptions=Index vector (dialog)  Indices=[3]  OutputSizes=1
  Sum : Sum  Inputs=|+-
  Sum1 : Sum  Inputs=|+++-
  Sum2 : Sum  Inputs=|+-
  Sum3 : Sum  Inputs=|+++-
  Sum4 : Sum  Inputs=|+++++
  Sum5 : Sum  Inputs=|+++++
  Transfer Fcn : TransferFcn  Numerator=[2*wc_pr 0]  Denominator=[1 2*wc_pr*wc_pr w_nom*w_nom]
  Transfer Fcn1 : TransferFcn  Numerator=[-K_h5*wc_hc 0]  Denominator=[1 2*wc_hc 5*w_nom*5*w_nom]
  Transfer Fcn10 : TransferFcn  Numerator=[-K_h9*wc_hc 0]  Denominator=[1 2*wc_hc 9*w_nom*9*w_nom]
  Transfer Fcn11 : TransferFcn  Numerator=[-K_h13*wc_hc 0]  Denominator=[1 2*wc_hc 13*w_nom*13*w_nom]
  Transfer Fcn2 : TransferFcn  Numerator=[2*wc_pr 0]  Denominator=[1 2*wc_pr*wc_pr w_nom*w_nom]
  Transfer Fcn3 : TransferFcn  Numerator=[-K_h7*wc_hc 0]  Denominator=[1 2*wc_hc 7*w_nom*7*w_nom]
  Transfer Fcn4 : TransferFcn  Numerator=[-K_h11*wc_hc 0]  Denominator=[1 2*wc_hc 11*w_nom*11*w_nom]
  Transfer Fcn5 : TransferFcn  Numerator=[-K_h5*wc_hc 0]  Denominator=[1 2*wc_hc 5*w_nom*5*w_nom]
  Transfer Fcn6 : TransferFcn  Numerator=[-K_h7*wc_hc 0]  Denominator=[1 2*wc_hc 7*w_nom*7*w_nom]
  Transfer Fcn7 : TransferFcn  Numerator=[-K_h9*wc_hc 0]  Denominator=[1 2*wc_hc 9*w_nom*9*w_nom]
  Transfer Fcn8 : TransferFcn  Numerator=[-K_h13*wc_hc 0]  Denominator=[1 2*wc_hc 13*w_nom*13*w_nom]
  Transfer Fcn9 : TransferFcn  Numerator=[-K_h11*wc_hc 0]  Denominator=[1 2*wc_hc 11*w_nom*11*w_nom]
  abc to Alpha-Beta-Zero : spsabctoAlphaBetaZeroLib/abc to Alpha-Beta-Zero
  abc to Alpha-Beta-Zero1 : spsabctoAlphaBetaZeroLib/abc to Alpha-Beta-Zero
  abc to Alpha-Beta-Zero2 : spsabctoAlphaBetaZeroLib/abc to Alpha-Beta-Zero
  Ref : Outport
  wires:
  Ref Voltage/1 -> abc to Alpha-Beta-Zero/1
  Selector/1 -> Sum/1
  Selector2/1 -> Sum/2
  Sum/1 -> Gain1/1, Transfer Fcn8/1, Transfer Fcn4/1, Transfer Fcn7/1, Transfer Fcn3/1, Transfer Fcn1/1, Gain/1
  Gain/1 -> Transfer Fcn/1
  Gain1/1 -> Sum1/1
  Transfer Fcn/1 -> Sum1/2
  Sum2/1 -> Gain3/1, Transfer Fcn11/1, Transfer Fcn9/1, Transfer Fcn10/1, Transfer Fcn6/1, Transfer Fcn5/1, Gain2/1
  Selector3/1 -> Sum2/1
  Gain2/1 -> Transfer Fcn2/1
  Transfer Fcn2/1 -> Sum3/2
  Gain3/1 -> Sum3/1
  abc to Alpha-Beta-Zero2/1 -> Selector6/1, Selector5/1
  Sum1/1 -> Mux/1
  Sum3/1 -> Mux/2
  Mux/1 -> Alpha-Beta-Zero to abc/1
  Inv current/1 -> abc to Alpha-Beta-Zero2/1
  Sum4/1 -> Sum1/3
  Transfer Fcn1/1 -> Sum4/1
  Transfer Fcn3/1 -> Sum4/2
  Transfer Fcn6/1 -> Sum5/2
  Selector4/1 -> Sum2/2
  Sum5/1 -> Sum3/3
  Transfer Fcn7/1 -> Sum4/3
  Transfer Fcn4/1 -> Sum4/4
  Transfer Fcn8/1 -> Sum4/5
  Transfer Fcn10/1 -> Sum5/3
  Transfer Fcn9/1 -> Sum5/4
  Transfer Fcn11/1 -> Sum5/5
  Selector6/1 -> Gain6/1
  Selector5/1 -> Gain5/1
  Transfer Fcn5/1 -> Sum5/1
  Selector7/1 -> Mux/3
  Gain5/1 -> Sum1/4
  Gain6/1 -> Sum3/4
  Load Voltage/1 -> abc to Alpha-Beta-Zero1/1
  abc to Alpha-Beta-Zero/1 -> Selector3/1, Selector/1
  abc to Alpha-Beta-Zero1/1 -> Selector4/1, Selector2/1
  Alpha-Beta-Zero to abc/1 -> Ref/1

== system Simulation_NoVI/Voltage Source Inverter 2/THD measurement ==
  In1 : Inport
  Demux : Demux  Outputs=3
  To Workspace : ToWorkspace  VariableName=phase1  SaveFormat=Structure With Time  SampleTime=-1
  To Workspace1 : ToWorkspace  VariableName=phase2  SaveFormat=Structure With Time  SampleTime=-1
  To Workspace2 : ToWorkspace  VariableName=phase3  SaveFormat=Structure With Time  SampleTime=-1
  wires:
  In1/1 -> Demux/1
  Demux/1 -> To Workspace/1
  Demux/2 -> To Workspace1/1
  Demux/3 -> To Workspace2/1

== system Simulation_NoVI/Voltage Source Inverter 2/dq converter ==
  Vodq : Inport
  Iodq : Inport  Port=2
  Ildq : Inport  Port=3
  wt : Inport  Port=4
  Scope : Scope
  Scope1 : Scope
  Subsystem : Subsystem
  Subsystem1 : Subsystem
  Subsystem2 : Subsystem
  Vod : Outport
  Voq : Outport  Port=2
  Iod : Outport  Port=3
  Ioq : Outport  Port=4
  Ild : Outport  Port=5
  Ilq : Outport  Port=6
  wires:
  Subsystem/1(Out1) -> Scope/1, Vod/1  "Vod"
  Subsystem1/1(Out1) -> Iod/1  "Iod"
  Subsystem/2(Out2) -> Voq/1  "Voq"
  wt/1 -> Subsystem2/2(wt), Subsystem1/2(wt), Subsystem/2(wt)
  Subsystem1/2(Out2) -> Ioq/1  "Ioq"
  Iodq/1 -> Subsystem1/1(abc)
  Subsystem2/2(Out2) -> Ilq/1  "Ilq"
  Ildq/1 -> Subsystem2/1(abc)
  Vodq/1 -> Subsystem/1(abc)
  Subsystem2/1(Out1) -> Scope1/1, Ild/1  "Vod"

== system Simulation_NoVI/Voltage Source Inverter 3/3to2 3 ==
  "single " : Inport
  "wt " : Inport  Port=2
  Add1 : Sum  Inputs=+++
  Constant2 : Constant  Value=2*pi/3
  Constant3 : Constant  Value=4*pi/3
  Constant4 : Constant  Value=exp(i*2*pi/3)
  Constant5 : Constant  Value=2/3
  Cos : Trigonometry  Operator=cos
  Cos1 : Trigonometry  Operator=cos
  Cos2 : Trigonometry  Operator=cos
  Math Function1 : Math  Operator=square  SignedPower=on
  Mux : Mux  Inputs=3
  Product{3..8} (6 alike) : Product  RndMeth=Zero
  Scope : Scope  NumInputPorts=3
  Sum : Sum  Inputs=|++
  Sum1 : Sum  Inputs=|++
  threePhase : Outport  VectorParamsAs1DForOutWhenUnconnected=off
  wires:
  "single "/1 -> Product5/1, Product4/1, Product3/1
  Cos/1 -> Product3/2
  Constant2/1 -> Sum/2
  Sum/1 -> Cos1/1
  Cos1/1 -> Product4/2
  "wt "/1 -> Sum1/1, Sum/1, Cos/1
  Constant3/1 -> Sum1/2
  Sum1/1 -> Cos2/1
  Cos2/1 -> Product5/2
  Constant4/1 -> Product7/1, Math Function1/1
  Product7/1 -> Add1/2
  Add1/1 -> Product6/1
  Product8/1 -> Add1/3
  Product5/1 -> Scope/3, Mux/3, Product8/2
  Product3/1 -> Scope/1, Mux/1, Add1/1
  Constant5/1 -> Product6/2
  Product4/1 -> Scope/2, Mux/2, Product7/2
  Math Function1/1 -> Product8/1
  Mux/1 -> threePhase/1

== system Simulation_NoVI/Voltage Source Inverter 3/Droop for secondary control2 ==
  P : Inport
  w_nom : Inport  Port=2
  V_nom : Inport  Port=3
  Q : Inport  Port=4
  Gain4 : Gain  Gain=n_q
  Gain5 : Gain  Gain=m_p
  Integrator : Integrator  WrapState=on  WrappedStateUpperValue=2*pi  WrappedStateLowerValue=0
  Sum1 : Sum  Inputs=|+-
  Sum2 : Sum  Inputs=|+-
  Vref : Outport
  wt : Outport  Port=2
  wo : Outport  Port=3
  wires:
  P/1 -> Gain5/1
  w_nom/1 -> Sum2/1
  Gain5/1 -> Sum2/2
  Sum2/1 -> wo/1, Integrator/1  "w"
  Integrator/1 -> wt/1
  V_nom/1 -> Sum1/1  "Vod_s"
  Gain4/1 -> Sum1/2
  Q/1 -> Gain4/1
  Sum1/1 -> Vref/1  "Vod_s"

== system Simulation_NoVI/Voltage Source Inverter 3/Low-pass filter ==
  p_hat : Inport
  q_hat : Inport  Port=2
  Low-Pass Filter (Discrete or Continuous) : eeGeneralControl/Low-Pass Filter (Discrete or Continuous)  K=1  T=lo_co  B=inf  A=-inf  init_option=Inherited from block input  x0=0  Ts=-1
  Low-Pass Filter (Discrete or Continuous)1 : eeGeneralControl/Low-Pass Filter (Discrete or Continuous)  K=1  T=lo_co  B=inf  A=-inf  init_option=Inherited from block input  x0=0  Ts=-1
  P : Outport
  Q : Outport  Port=2
  wires:
  q_hat/1 -> Low-Pass Filter (Discrete or Continuous)1/1
  Low-Pass Filter (Discrete or Continuous)1/1 -> Q/1  "Q"
  Low-Pass Filter (Discrete or Continuous)/1 -> P/1  "P"
  p_hat/1 -> Low-Pass Filter (Discrete or Continuous)/1

== system Simulation_NoVI/Voltage Source Inverter 3/PLL_1p1 ==
  v : Inport
  2pi : Constant  Value=2*pi
  Low-Pass Filter (Discrete or Continuous) : eeGeneralControl/Low-Pass Filter (Discrete or Continuous)  K=1  T=lo_co  B=inf  A=-inf  init_option=Inherited from block input  x0=0  Ts=-1
  PID Controller : slpidlib/PID Controller  Controller=PI  Form=Parallel  TimeDomain=Continuous-time  UseExternalTs=off  SampleTime=-1  IntegratorMethod=Forward Euler  FilterMethod=Forward Euler  ControllerParametersSource=internal  P=100.15925  I=9869  UseKiTs=off  D=0  N=100  UseFilter=on  TunerSelectOption=Transfer Function Based (PID Tuner App)  InitialConditionSource=internal  InitialConditionForIntegrator=0  InitialConditionForFilter=0  DifferentiatorICPrevScaledInput=0  ExternalReset=none  TrackingMode=off  Kt=1  LimitOutput=off  SatLimitsSource=internal  UpperSaturationLimit=inf  LowerSaturationLimit=-inf  LinearizeAsGain=off  AntiWindupMode=none  Kb=1  LimitIntegrator=off  UpperIntegratorSaturationLimit=inf  LowerIntegratorSaturationLimit=-inf  POutMin=[]  POutMax=[]  IOutMin=[]  IOutMax=[]  DOutMin=[]  DOutMax=[]  NOutMin=[]  NOutMax=[]  SumOutMin=[]  SumOutMax=[]  SaturationOutMin=[]  SaturationOutMax=[]  PParamMin=[]  PParamMax=[]  IParamMin=[]  IParamMax=[]  DParamMin=[]  DParamMax=[]  NParamMin=[]  NParamMax=[]  KbParamMin=[]  KbParamMax=[]  KtParamMin=[]  KtParamMax=[]  KbOutMin=[]  KbOutMax=[]  KtOutMin=[]  KtOutMax=[]  IntegratorOutMin=[]  IntegratorOutMax=[]  FilterOutMin=[]  FilterOutMax=[]  SumI1OutMin=[]  SumI1OutMax=[]  SumI2OutMin=[]  SumI2OutMax=[]  SumI3OutMin=[]  SumI3OutMax=[]  SumI4OutMin=[]  SumI4OutMax=[]  SumDOutMin=[]  SumDOutMax=[]  DifferentiatorOutMin=[]  DifferentiatorOutMax=[]  FilterDiffOutCoefMin=[]  FilterDiffOutCoefMax=[]  ReciprocalOutMin=[]  ReciprocalOutMax=[]  SumDenOutMin=[]  SumDenOutMax=[]  SumNumOutMin=[]  SumNumOutMax=[]  DivideOutMin=[]  DivideOutMax=[]  UdiffTsProdOutMin=[]  UdiffTsProdOutMax=[]  NTsProdOutMin=[]  NTsProdOutMax=[]  UintegralTsProdOutMin=[]  UintegralTsProdOutMax=[]  UngainTsProdOutMin=[]  UngainTsProdOutMax=[]  ClampingZeroOutDataTypeStr=Inherit: Inherit via back propagation  ClampingZeroOutMin=[]  ClampingZeroOutMax=[]  FilterDenConstantOutDataTypeStr=Inherit: Inherit via back propagation  FilterDenConstantOutMin=[]  FilterDenConstantOutMax=[]  PCopyOutDataTypeStr=Inherit: Inherit via back propagation  PCopyOutMin=[]  PCopyOutMax=[]  NCopyOutDataTypeStr=Inherit: Inherit via back propagation  NCopyOutMin=[]  NCopyOutMax=[]  IntegratorContinuousStateAttributes=''  IntegratorStateMustResolveToSignalObject=off  IntegratorRTWStateStorageClass=Auto  FilterContinuousStateAttributes=''  FilterStateMustResolveToSignalObject=off  FilterRTWStateStorageClass=Auto  ParallelPVariant=InternalParameters  IdealPVariant=Disabled  IVariant=InternalParameters  DVariant=Disabled  IntegratorVariant=Continuous  SatVariant=Disabled  AWVariant=Passthrough  PCopyVariant=Disabled  TRVariant=Disabled  FdbkBlocksVariant=Forward  IdealPFdbkVariant=Disabled  SatFdbkVariant=Disabled  DerivativeFilterVariant=Disabled  NVariant=Disabled  NCopyVariant=Disabled_SignalSpec  FilterICVariant=Disabled  IntegratorICVariant=InternalICs  ExternalResetVariant=Disabled  TRSumVariant=Passthrough  SumFdbkVariant=Disabled  SumVariant=Sum_PI  TsampFilterVariant=InternalTs  TsampNgainVariant=Passthrough  TsampIntegralVariant=Passthrough  ExternalSaturationOutDataTypeStr=Inherit: Same as second input
  Reset1 : RelationalOperator  OutDataTypeStr=boolean  InputSameDT=off
  Scope : Scope
  Sqrt : Sqrt
  Square : Math  Operator=square
  Square1 : Math  Operator=square
  Sum : Sum  Inputs=|++
  Sum1 : Sum  Inputs=|++
  TienXuly : Subsystem  mask{k=0.5, fc1=50, fc2=10}
      mask prompts: k "he so k"; fc1 "Tan so cat cua bo loc bac 2"; fc2 "Tan so cat cua bo loc thong thap"
  Tinhtheta : Integrator  ExternalReset=rising  UpperSaturationLimit=2*pi
  apha-beta=>dq : Subsystem
  wff : Constant  Value=50*2*pi
  v_dq : Outport
  omega : Outport  Port=2
  wires:
  PID Controller/1 -> Sum1/1
  v/1 -> TienXuly/1(v)
  Tinhtheta/1 -> apha-beta=>dq/1(Theta), Reset1/1
  TienXuly/2(v'q) -> apha-beta=>dq/3(Ubeta)
  apha-beta=>dq/1(vq) -> Square1/1, PID Controller/1
  TienXuly/1(v') -> apha-beta=>dq/2(Uapha)
  2pi/1 -> Reset1/2
  wff/1 -> Sum1/2
  Reset1/1 -> Tinhtheta/2
  apha-beta=>dq/2(vd) -> Square/1
  Square/1 -> Sum/1
  Square1/1 -> Sum/2
  Sum/1 -> Sqrt/1
  Sqrt/1 -> v_dq/1
  Sum1/1 -> Low-Pass Filter (Discrete or Continuous)/1, Tinhtheta/1  "P"
  Low-Pass Filter (Discrete or Continuous)/1 -> Scope/1, omega/1  "P"

== system Simulation_NoVI/Voltage Source Inverter 3/PLL_1p2 ==
  v : Inport
  2pi : Constant  Value=2*pi
  Low-Pass Filter (Discrete or Continuous) : eeGeneralControl/Low-Pass Filter (Discrete or Continuous)  K=1  T=lo_co  B=inf  A=-inf  init_option=Inherited from block input  x0=0  Ts=-1
  PID Controller : slpidlib/PID Controller  Controller=PI  Form=Parallel  TimeDomain=Continuous-time  UseExternalTs=off  SampleTime=-1  IntegratorMethod=Forward Euler  FilterMethod=Forward Euler  ControllerParametersSource=internal  P=100.15925  I=9869  UseKiTs=off  D=0  N=100  UseFilter=on  TunerSelectOption=Transfer Function Based (PID Tuner App)  InitialConditionSource=internal  InitialConditionForIntegrator=0  InitialConditionForFilter=0  DifferentiatorICPrevScaledInput=0  ExternalReset=none  TrackingMode=off  Kt=1  LimitOutput=off  SatLimitsSource=internal  UpperSaturationLimit=inf  LowerSaturationLimit=-inf  LinearizeAsGain=off  AntiWindupMode=none  Kb=1  LimitIntegrator=off  UpperIntegratorSaturationLimit=inf  LowerIntegratorSaturationLimit=-inf  POutMin=[]  POutMax=[]  IOutMin=[]  IOutMax=[]  DOutMin=[]  DOutMax=[]  NOutMin=[]  NOutMax=[]  SumOutMin=[]  SumOutMax=[]  SaturationOutMin=[]  SaturationOutMax=[]  PParamMin=[]  PParamMax=[]  IParamMin=[]  IParamMax=[]  DParamMin=[]  DParamMax=[]  NParamMin=[]  NParamMax=[]  KbParamMin=[]  KbParamMax=[]  KtParamMin=[]  KtParamMax=[]  KbOutMin=[]  KbOutMax=[]  KtOutMin=[]  KtOutMax=[]  IntegratorOutMin=[]  IntegratorOutMax=[]  FilterOutMin=[]  FilterOutMax=[]  SumI1OutMin=[]  SumI1OutMax=[]  SumI2OutMin=[]  SumI2OutMax=[]  SumI3OutMin=[]  SumI3OutMax=[]  SumI4OutMin=[]  SumI4OutMax=[]  SumDOutMin=[]  SumDOutMax=[]  DifferentiatorOutMin=[]  DifferentiatorOutMax=[]  FilterDiffOutCoefMin=[]  FilterDiffOutCoefMax=[]  ReciprocalOutMin=[]  ReciprocalOutMax=[]  SumDenOutMin=[]  SumDenOutMax=[]  SumNumOutMin=[]  SumNumOutMax=[]  DivideOutMin=[]  DivideOutMax=[]  UdiffTsProdOutMin=[]  UdiffTsProdOutMax=[]  NTsProdOutMin=[]  NTsProdOutMax=[]  UintegralTsProdOutMin=[]  UintegralTsProdOutMax=[]  UngainTsProdOutMin=[]  UngainTsProdOutMax=[]  ClampingZeroOutDataTypeStr=Inherit: Inherit via back propagation  ClampingZeroOutMin=[]  ClampingZeroOutMax=[]  FilterDenConstantOutDataTypeStr=Inherit: Inherit via back propagation  FilterDenConstantOutMin=[]  FilterDenConstantOutMax=[]  PCopyOutDataTypeStr=Inherit: Inherit via back propagation  PCopyOutMin=[]  PCopyOutMax=[]  NCopyOutDataTypeStr=Inherit: Inherit via back propagation  NCopyOutMin=[]  NCopyOutMax=[]  IntegratorContinuousStateAttributes=''  IntegratorStateMustResolveToSignalObject=off  IntegratorRTWStateStorageClass=Auto  FilterContinuousStateAttributes=''  FilterStateMustResolveToSignalObject=off  FilterRTWStateStorageClass=Auto  ParallelPVariant=InternalParameters  IdealPVariant=Disabled  IVariant=InternalParameters  DVariant=Disabled  IntegratorVariant=Continuous  SatVariant=Disabled  AWVariant=Passthrough  PCopyVariant=Disabled  TRVariant=Disabled  FdbkBlocksVariant=Forward  IdealPFdbkVariant=Disabled  SatFdbkVariant=Disabled  DerivativeFilterVariant=Disabled  NVariant=Disabled  NCopyVariant=Disabled_SignalSpec  FilterICVariant=Disabled  IntegratorICVariant=InternalICs  ExternalResetVariant=Disabled  TRSumVariant=Passthrough  SumFdbkVariant=Disabled  SumVariant=Sum_PI  TsampFilterVariant=InternalTs  TsampNgainVariant=Passthrough  TsampIntegralVariant=Passthrough  ExternalSaturationOutDataTypeStr=Inherit: Same as second input
  Reset1 : RelationalOperator  OutDataTypeStr=boolean  InputSameDT=off
  Scope : Scope
  Sqrt : Sqrt
  Square : Math  Operator=square
  Square1 : Math  Operator=square
  Sum : Sum  Inputs=|++
  Sum1 : Sum  Inputs=|++
  TienXuly : Subsystem  mask{k=0.5, fc1=50, fc2=10}
      mask prompts: k "he so k"; fc1 "Tan so cat cua bo loc bac 2"; fc2 "Tan so cat cua bo loc thong thap"
  Tinhtheta : Integrator  ExternalReset=rising  UpperSaturationLimit=2*pi
  apha-beta=>dq : Subsystem
  wff : Constant  Value=50*2*pi
  v_dq : Outport
  omega : Outport  Port=2
  wires:
  PID Controller/1 -> Sum1/1
  v/1 -> TienXuly/1(v)
  Tinhtheta/1 -> apha-beta=>dq/1(Theta), Reset1/1
  TienXuly/2(v'q) -> apha-beta=>dq/3(Ubeta)
  apha-beta=>dq/1(vq) -> Square1/1, PID Controller/1
  TienXuly/1(v') -> apha-beta=>dq/2(Uapha)
  2pi/1 -> Reset1/2
  wff/1 -> Sum1/2
  Reset1/1 -> Tinhtheta/2
  apha-beta=>dq/2(vd) -> Square/1
  Square/1 -> Sum/1
  Square1/1 -> Sum/2
  Sum/1 -> Sqrt/1
  Sqrt/1 -> v_dq/1
  Sum1/1 -> Low-Pass Filter (Discrete or Continuous)/1, Tinhtheta/1  "P"
  Low-Pass Filter (Discrete or Continuous)/1 -> Scope/1, omega/1  "P"

== system Simulation_NoVI/Voltage Source Inverter 3/PMW ==
  REF : Inport
  Tri_signal : Inport  Port=2
  Demux : Demux  Outputs=3
  Mux : Mux  Inputs=6
  NOT : Logic  Operator=NOT  AllPortsSameDT=off  OutDataTypeStr=boolean
  NOT1 : Logic  Operator=NOT  AllPortsSameDT=off  OutDataTypeStr=boolean
  NOT2 : Logic  Operator=NOT  AllPortsSameDT=off  OutDataTypeStr=boolean
  Relational Operator : RelationalOperator  OutDataTypeStr=boolean  RndMeth=Simplest  InputSameDT=off
  Relational Operator1 : RelationalOperator  OutDataTypeStr=boolean  RndMeth=Simplest  InputSameDT=off
  Relational Operator2 : RelationalOperator  OutDataTypeStr=boolean  RndMeth=Simplest  InputSameDT=off
  Scope : Scope
  Scope1 : Scope
  Scope2 : Scope  NumInputPorts=2
  Out1 : Outport
  wires:
  Demux/1 -> Relational Operator/1
  Tri_signal/1 -> Relational Operator1/2, Relational Operator/2, Relational Operator2/2
  Demux/2 -> Relational Operator1/1
  Demux/3 -> Relational Operator2/1
  REF/1 -> Scope1/1, Demux/1
  Relational Operator/1 -> Scope2/1, Mux/1, NOT/1
  NOT/1 -> Scope2/2, Mux/2
  Relational Operator1/1 -> NOT1/1, Mux/3
  NOT1/1 -> Mux/4
  Relational Operator2/1 -> Mux/5, NOT2/1
  NOT2/1 -> Mux/6
  Mux/1 -> Scope/1, Out1/1

== system Simulation_NoVI/Voltage Source Inverter 3/PQ calculator ==
  Vod : Inport
  Voq : Inport  Port=2
  Iod : Inport  Port=3
  Ioq : Inport  Port=4
  Product{,1..3} (4 alike) : Product
  Scope : Scope
  Sum10 : Sum  Inputs=|++
  Sum11 : Sum  Inputs=|+-
  p_hat : Outport
  q_hat : Outport  Port=2
  wires:
  Product3/1 -> Sum11/2
  Product1/1 -> Sum10/2
  Voq/1 -> Product3/1, Product1/1
  Iod/1 -> Product/2, Product3/2
  Product2/1 -> Sum11/1
  Ioq/1 -> Product1/2, Product2/2
  Product/1 -> Sum10/1
  Vod/1 -> Scope/1, Product/1, Product2/1
  Sum11/1 -> q_hat/1  "q_hat"
  Sum10/1 -> p_hat/1  "p_hat"

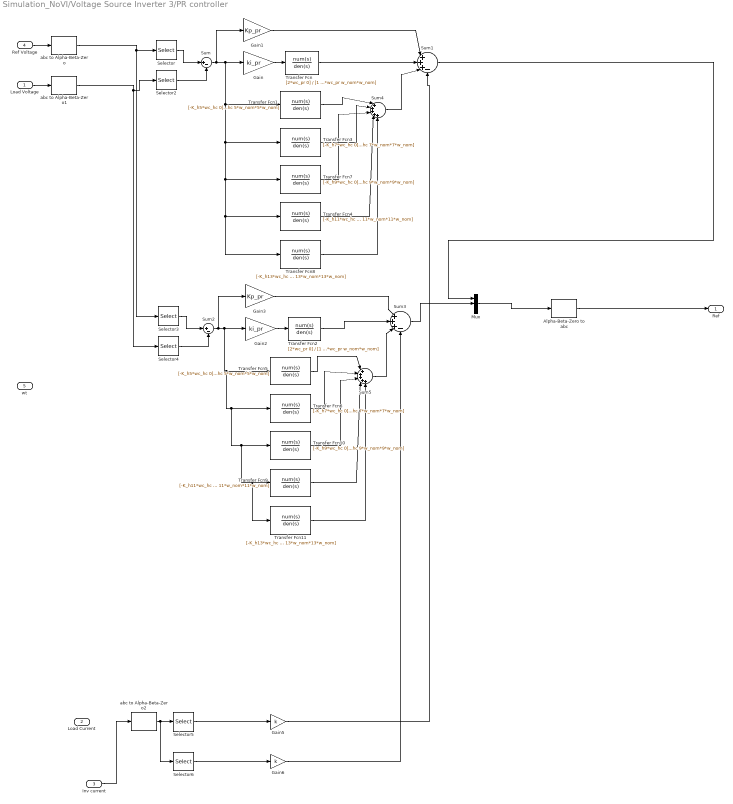
== system Simulation_NoVI/Voltage Source Inverter 3/PR controller ==
  Load Voltage : Inport
  Load Current : Inport  Port=2
  Inv current : Inport  Port=3
  Ref Voltage : Inport  Port=4
  wt : Inport  Port=5
  Alpha-Beta-Zero to abc : spsAlphaBetaZerotoabcLib/Alpha-Beta-Zero to abc
      settings: LibrarySourceBlock=|
      | sps_lib/Control/Alpha-Beta-Zero
      | to abc
  Gain : Gain  Gain=ki_pr
  Gain1 : Gain  Gain=Kp_pr
  Gain2 : Gain  Gain=ki_pr
  Gain3 : Gain  Gain=Kp_pr
  Gain5 : Gain  Gain=k
  Gain6 : Gain  Gain=k
  Mux : Mux  Inputs=3
  Selector : Selector  InputPortWidth=3  IndexOptions=Index vector (dialog)  Indices=[1]  OutputSizes=1
  Selector2 : Selector  InputPortWidth=3  IndexOptions=Index vector (dialog)  Indices=[1]  OutputSizes=1
  Selector3 : Selector  InputPortWidth=3  IndexOptions=Index vector (dialog)  Indices=[2]  OutputSizes=1
  Selector4 : Selector  InputPortWidth=3  IndexOptions=Index vector (dialog)  Indices=[2]  OutputSizes=1
  Selector5 : Selector  InputPortWidth=3  IndexOptions=Index vector (dialog)  Indices=[1]  OutputSizes=1
  Selector6 : Selector  InputPortWidth=3  IndexOptions=Index vector (dialog)  Indices=[2]  OutputSizes=1
  Sum : Sum  Inputs=|+-
  Sum1 : Sum  Inputs=|+++-
  Sum2 : Sum  Inputs=|+-
  Sum3 : Sum  Inputs=|+++-
  Sum4 : Sum  Inputs=|+++++
  Sum5 : Sum  Inputs=|+++++
  Transfer Fcn : TransferFcn  Numerator=[2*wc_pr 0]  Denominator=[1 2*wc_pr*wc_pr w_nom*w_nom]
  Transfer Fcn1 : TransferFcn  Numerator=[-K_h5*wc_hc 0]  Denominator=[1 2*wc_hc 5*w_nom*5*w_nom]
  Transfer Fcn10 : TransferFcn  Numerator=[-K_h9*wc_hc 0]  Denominator=[1 2*wc_hc 9*w_nom*9*w_nom]
  Transfer Fcn11 : TransferFcn  Numerator=[-K_h13*wc_hc 0]  Denominator=[1 2*wc_hc 13*w_nom*13*w_nom]
  Transfer Fcn2 : TransferFcn  Numerator=[2*wc_pr 0]  Denominator=[1 2*wc_pr*wc_pr w_nom*w_nom]
  Transfer Fcn3 : TransferFcn  Numerator=[-K_h7*wc_hc 0]  Denominator=[1 2*wc_hc 7*w_nom*7*w_nom]
  Transfer Fcn4 : TransferFcn  Numerator=[-K_h11*wc_hc 0]  Denominator=[1 2*wc_hc 11*w_nom*11*w_nom]
  Transfer Fcn5 : TransferFcn  Numerator=[-K_h5*wc_hc 0]  Denominator=[1 2*wc_hc 5*w_nom*5*w_nom]
  Transfer Fcn6 : TransferFcn  Numerator=[-K_h7*wc_hc 0]  Denominator=[1 2*wc_hc 7*w_nom*7*w_nom]
  Transfer Fcn7 : TransferFcn  Numerator=[-K_h9*wc_hc 0]  Denominator=[1 2*wc_hc 9*w_nom*9*w_nom]
  Transfer Fcn8 : TransferFcn  Numerator=[-K_h13*wc_hc 0]  Denominator=[1 2*wc_hc 13*w_nom*13*w_nom]
  Transfer Fcn9 : TransferFcn  Numerator=[-K_h11*wc_hc 0]  Denominator=[1 2*wc_hc 11*w_nom*11*w_nom]
  abc to Alpha-Beta-Zero : spsabctoAlphaBetaZeroLib/abc to Alpha-Beta-Zero
  abc to Alpha-Beta-Zero1 : spsabctoAlphaBetaZeroLib/abc to Alpha-Beta-Zero
  abc to Alpha-Beta-Zero2 : spsabctoAlphaBetaZeroLib/abc to Alpha-Beta-Zero
  Ref : Outport
  wires:
  Ref Voltage/1 -> abc to Alpha-Beta-Zero/1
  Selector/1 -> Sum/1
  Selector2/1 -> Sum/2
  Sum/1 -> Gain1/1, Transfer Fcn8/1, Transfer Fcn4/1, Transfer Fcn7/1, Transfer Fcn3/1, Transfer Fcn1/1, Gain/1
  Gain/1 -> Transfer Fcn/1
  Gain1/1 -> Sum1/1
  Transfer Fcn/1 -> Sum1/2
  Sum2/1 -> Gain3/1, Transfer Fcn11/1, Transfer Fcn9/1, Transfer Fcn10/1, Transfer Fcn6/1, Transfer Fcn5/1, Gain2/1
  Selector3/1 -> Sum2/1
  Gain2/1 -> Transfer Fcn2/1
  Transfer Fcn2/1 -> Sum3/2
  Gain3/1 -> Sum3/1
  abc to Alpha-Beta-Zero2/1 -> Selector6/1, Selector5/1
  Sum1/1 -> Mux/1
  Sum3/1 -> Mux/2
  Mux/1 -> Alpha-Beta-Zero to abc/1
  Inv current/1 -> abc to Alpha-Beta-Zero2/1
  Sum4/1 -> Sum1/3
  Transfer Fcn1/1 -> Sum4/1
  Transfer Fcn3/1 -> Sum4/2
  Transfer Fcn6/1 -> Sum5/2
  Selector4/1 -> Sum2/2
  Sum5/1 -> Sum3/3
  Transfer Fcn7/1 -> Sum4/3
  Transfer Fcn4/1 -> Sum4/4
  Transfer Fcn8/1 -> Sum4/5
  Transfer Fcn10/1 -> Sum5/3
  Transfer Fcn9/1 -> Sum5/4
  Transfer Fcn11/1 -> Sum5/5
  Selector6/1 -> Gain6/1
  Selector5/1 -> Gain5/1
  Transfer Fcn5/1 -> Sum5/1
  Gain5/1 -> Sum1/4
  Gain6/1 -> Sum3/4
  Load Voltage/1 -> abc to Alpha-Beta-Zero1/1
  abc to Alpha-Beta-Zero/1 -> Selector3/1, Selector/1
  abc to Alpha-Beta-Zero1/1 -> Selector4/1, Selector2/1
  Alpha-Beta-Zero to abc/1 -> Ref/1

== system Simulation_NoVI/Voltage Source Inverter 3/dq converter ==
  Vodq : Inport
  Iodq : Inport  Port=2
  Ildq : Inport  Port=3
  wt : Inport  Port=4
  Scope : Scope
  Scope1 : Scope
  Subsystem : Subsystem
  Subsystem1 : Subsystem
  Subsystem2 : Subsystem
  Vod : Outport
  Voq : Outport  Port=2
  Iod : Outport  Port=3
  Ioq : Outport  Port=4
  Ild : Outport  Port=5
  Ilq : Outport  Port=6
  wires:
  Subsystem/1(Out1) -> Scope/1, Vod/1  "Vod"
  Subsystem1/1(Out1) -> Iod/1  "Iod"
  Subsystem/2(Out2) -> Voq/1  "Voq"
  wt/1 -> Subsystem2/2(wt), Subsystem1/2(wt), Subsystem/2(wt)
  Subsystem1/2(Out2) -> Ioq/1  "Ioq"
  Iodq/1 -> Subsystem1/1(abc)
  Subsystem2/2(Out2) -> Ilq/1  "Ilq"
  Ildq/1 -> Subsystem2/1(abc)
  Vodq/1 -> Subsystem/1(abc)
  Subsystem2/1(Out1) -> Scope1/1, Ild/1  "Vod"
